simulink model "SegwayLinearized0Controlled"  (R2019a)
settings: Solver=VariableStepAuto  StartTime=0.0  StopTime=10.0  RelTol=1e-3
undefined symbols (not defined in the file): A, B, C, D, K, X0lin0
settings Model: Creator=Huynh  LastModifiedBy=Huynh

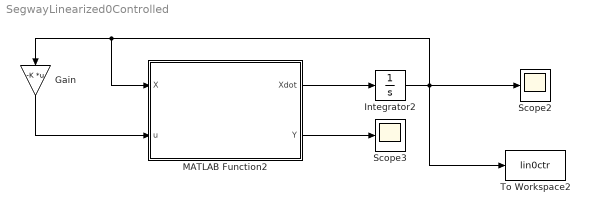
== system SegwayLinearized0Controlled ==
  Gain : Gain  Gain=-K  Multiplication=Matrix(K*u)
  Integrator2 : Integrator  InitialCondition=X0lin0
  MATLAB Function2 : MATLAB Function  TreatAsAtomicUnit=on
  Scope2 : Scope
  Scope3 : Scope
  To Workspace2 : ToWorkspace  VariableName=lin0ctr  SampleTime=-1
  wires:
  Integrator2/1 -> Gain/1, MATLAB Function2/1(X), To Workspace2/1, Scope2/1
  MATLAB Function2/1(Xdot) -> Integrator2/1
  Gain/1 -> MATLAB Function2/2(u)
  MATLAB Function2/2(Y) -> Scope3/1

== matlab function SegwayLinearized0Controlled/MATLAB Function2 ==
  data: X input; Xdot output; A parameter; B parameter; C parameter; D parameter; Y output; u input
function [Xdot, Y] = LinearZeroSegway(X, A, B, C, D, u)
Xdot = A * X + B * u;
Y = C*X + D*u;
end
